simulink model "Simulation"  (R2019a)
settings: Solver=ode4  StartTime=0.0  StopTime=10  FixedStep=Ts  RelTol=1e-3
values from neighbouring files (symbols this model uses):
  B = (A'*A)\(A'*(Km*I)')    [Parametros_motor.m]
  J = M*R_rueda^2    (= 0.002772225)    [Parametros_motor.m]
  K = lqr(A_mat,B_mat,Q,R_mat)    [Parametros_motor.m]
  Ke = Ke'    [Parametros_motor.m]
  Km = (A'*A)\(A'*E')    [Parametros_motor.m]
  L = 2.04e-3    (= 0.00204)    [Parametros_motor.m]
  R = 5.06    [Parametros_motor.m]
  Ts = 1e-5    (= 1e-05)    [Parametros_motor.m]
  Tsc = 1e-3    (= 0.001)    [Parametros_motor.m]
  Tsco = 1e-3    (= 0.001)    [Parametros_motor.m]
undefined symbols (not defined in the file or in its folder): DiscIntNeverNeededParam
settings Model: SimulationMode=accelerator  Creator=cordo  LastModifiedBy=User

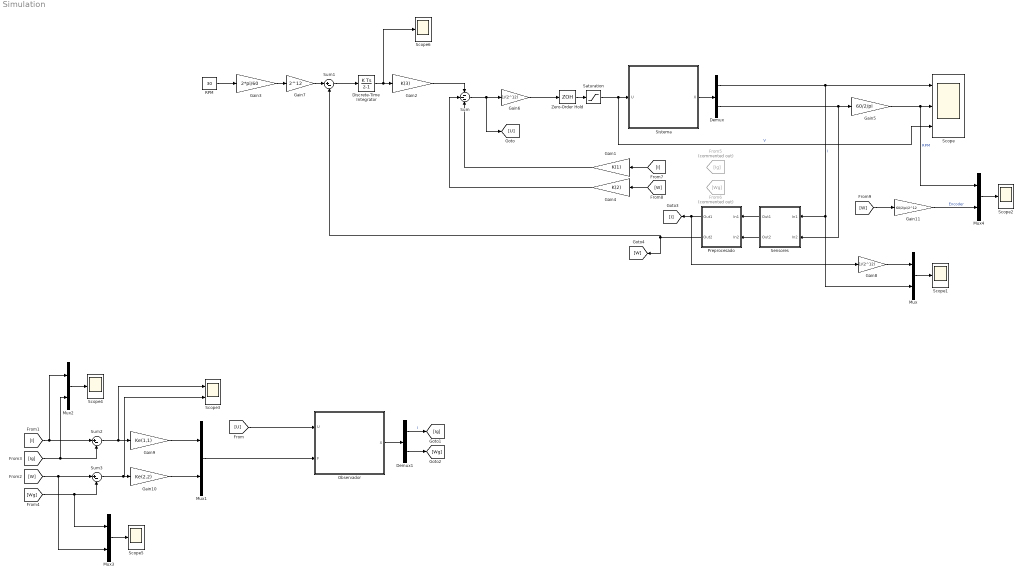
== system Simulation ==
  Demux : Demux  Outputs=2
  Demux1 : Demux  Outputs=2
  Discrete-Time Integrator : DiscreteIntegrator  SampleTime=Tsc  ICPrevOutput=DiscIntNeverNeededParam  ICPrevScaledInput=DiscIntNeverNeededParam
  From5 : From  Commented=on  GotoTag=Ig
  From6 : From  Commented=on  GotoTag=Wg
  Gain1 : Gain  Gain=K(1)
  Gain10 : Gain  Gain=Ke(2,2)
  Gain11 : Gain  Gain=60/2/pi/2^12
  Gain2 : Gain  Gain=K(3)
  Gain3 : Gain  Gain=2*pi/60
  Gain4 : Gain  Gain=K(2)
  Gain5 : Gain  Gain=60/2/pi
  Gain6 : Gain  Gain=1/(2^12)
  Gain7 : Gain  Gain=2^12
  Gain8 : Gain  Gain=1/(2^12)
  Gain9 : Gain  Gain=Ke(1,1)
  Mux{,1..4} (5 alike) : Mux  Inputs=2
  Observador : Subsystem
  Preprocesado : Subsystem
  RPM : Constant  Value=30  SampleTime=Ts
  Saturation : Saturate  UpperLimit=12.8  LowerLimit=-12.8
  Scope : Scope  NumInputPorts=3
  Scope{1..2,4..6} (5 alike) : Scope
  Scope3 : Scope  NumInputPorts=2
  Sensores : Subsystem
  Sistema : Subsystem
  Sum : Sum  Inputs=---
  Sum1 : Sum  Inputs=|+-
  Sum2 : Sum  Inputs=|+-
  Sum3 : Sum  Inputs=|+-
  Zero-Order Hold : ZeroOrderHold  SampleTime=Tsc
  wires:
  Sistema/1(X) -> Demux/1
  Demux/2 -> Sensores/2(In2), Gain5/1
  Demux/1 -> Mux/2, Sensores/1(In1), Scope/1  "I"
  Discrete-Time Integrator/1 -> Scope6/1, Gain2/1
  Gain4/1 -> Sum/2
  Gain3/1 -> Gain7/1
  RPM/1 -> Gain3/1
  Gain2/1 -> Sum/1
  Gain5/1 -> Mux4/1, Scope/2  "RPM"
  Sum/1 -> [U], Gain6/1
  Zero-Order Hold/1 -> Saturation/1
  Saturation/1 -> Scope/3, Sistema/1(U)  "V"
  Sum1/1 -> Discrete-Time Integrator/1
  Sensores/1(Out1) -> Preprocesado/1(In1)
  Sensores/2(Out2) -> Preprocesado/2(In2)
  Mux/1 -> Scope1/1
  Preprocesado/1(Out1) -> [I], Gain8/1
  Preprocesado/2(Out2) -> Sum1/2, [W]
  Gain6/1 -> Zero-Order Hold/1
  Gain7/1 -> Sum1/1
  Gain8/1 -> Mux/1
  Mux1/1 -> Observador/2(F)
  Gain9/1 -> Mux1/1
  Gain10/1 -> Mux1/2
  Observador/1(X) -> Demux1/1
  Demux1/1 -> [Ig]  "I"
  Demux1/2 -> [Wg]
  Sum2/1 -> Scope3/1, Gain9/1
  [I] -> Mux2/1, Sum2/1
  Sum3/1 -> Scope3/2, Gain10/1
  [Ig] -> Mux2/2, Sum2/2
  [Wg] -> Mux3/1, Sum3/2
  [U] -> Observador/1(U)
  Mux2/1 -> Scope4/1
  Mux3/1 -> Scope5/1
  [W] -> Mux3/2, Sum3/1
  [I] -> Gain1/1
  [W] -> Gain4/1
  Mux4/1 -> Scope2/1
  [W] -> Gain11/1
  Gain11/1 -> Mux4/2  "Encoder"
  Gain1/1 -> Sum/3

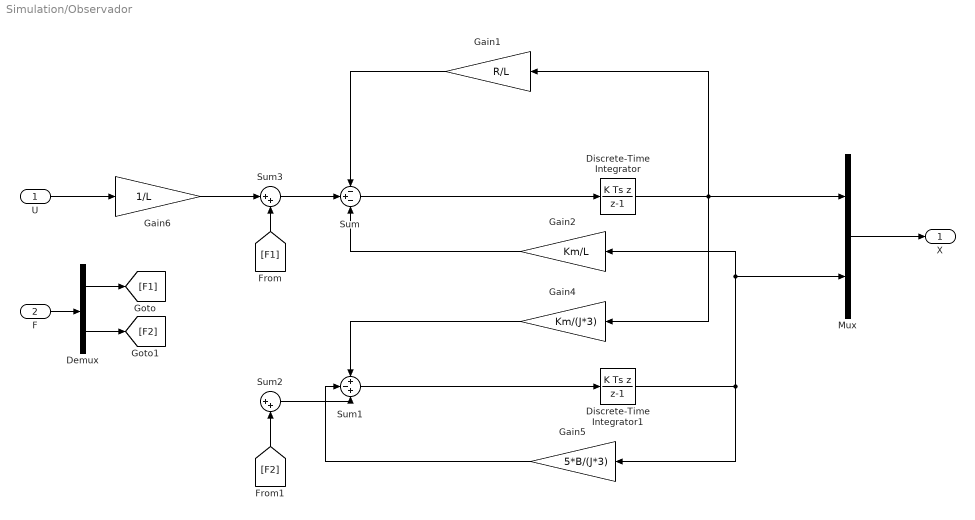
== system Simulation/Observador ==
  U : Inport
  F : Inport  Port=2
  Demux : Demux  Outputs=2
  Discrete-Time Integrator : DiscreteIntegrator  IntegratorMethod=Integration: Backward Euler  SampleTime=Tsco  ICPrevOutput=DiscIntNeverNeededParam  ICPrevScaledInput=DiscIntNeverNeededParam
  Discrete-Time Integrator1 : DiscreteIntegrator  IntegratorMethod=Integration: Backward Euler  SampleTime=Tsco  ICPrevOutput=DiscIntNeverNeededParam  ICPrevScaledInput=DiscIntNeverNeededParam
  Gain1 : Gain  Gain=R/L
  Gain2 : Gain  Gain=Km/L
  Gain4 : Gain  Gain=Km/(J*3)
  Gain5 : Gain  Gain=5*B/(J*3)
  Gain6 : Gain  Gain=1/L
  Mux : Mux  Inputs=2
  Sum : Sum  Inputs=-+-
  Sum1 : Sum  Inputs=+-+
  Sum2 : Sum  Inputs=|++
  Sum3 : Sum  Inputs=|++
  X : Outport
  wires:
  U/1 -> Gain6/1
  Mux/1 -> X/1
  Discrete-Time Integrator/1 -> Mux/1, Gain4/1, Gain1/1
  Sum1/1 -> Discrete-Time Integrator1/1
  Discrete-Time Integrator1/1 -> Mux/2, Gain2/1, Gain5/1
  Sum/1 -> Discrete-Time Integrator/1
  Gain2/1 -> Sum/3
  Gain4/1 -> Sum1/1
  Gain1/1 -> Sum/1
  Gain5/1 -> Sum1/2
  Sum2/1 -> Sum1/3
  Sum3/1 -> Sum/2
  Gain6/1 -> Sum3/1
  F/1 -> Demux/1
  Demux/1 -> [F1]
  [F1] -> Sum3/2
  Demux/2 -> [F2]
  [F2] -> Sum2/2

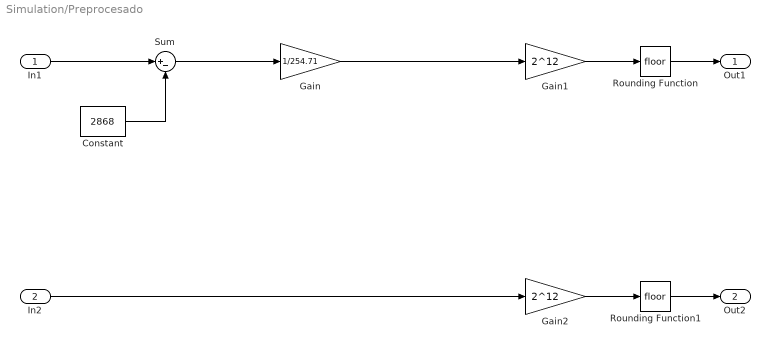
== system Simulation/Preprocesado ==
  In1 : Inport
  In2 : Inport  Port=2
  Constant : Constant  Value=2868
  Gain : Gain  Gain=1/254.71
  Gain1 : Gain  Gain=2^12
  Gain2 : Gain  Gain=2^12
  Rounding Function : Rounding
  Rounding Function1 : Rounding
  Sum : Sum  Inputs=|+-
  Out1 : Outport
  Out2 : Outport  Port=2
  wires:
  In2/1 -> Gain2/1
  Constant/1 -> Sum/2
  Sum/1 -> Gain/1
  In1/1 -> Sum/1
  Gain/1 -> Gain1/1
  Gain1/1 -> Rounding Function/1
  Gain2/1 -> Rounding Function1/1
  Rounding Function/1 -> Out1/1
  Rounding Function1/1 -> Out2/1

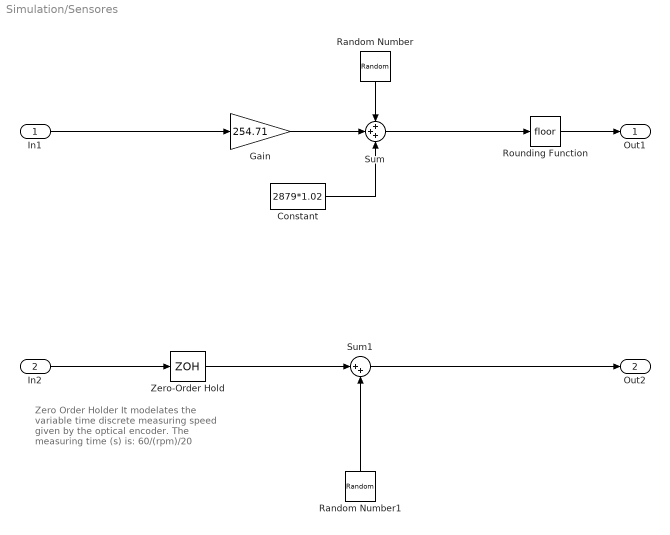
== system Simulation/Sensores ==
  note: Zero Order Holder
      | It modelates the variable time discrete
      | measuring  speed given by the optical
      | encoder.
      |
      | The measuring time (s) is:
      |
      | 60/(rpm)/20
  In1 : Inport
  In2 : Inport  Port=2
  Constant : Constant  Value=2879*1.02
  Gain : Gain  Gain=254.71
  Random Number : RandomNumber  Variance=20^2  SampleTime=Tsc
  Random Number1 : RandomNumber  Variance=4  SampleTime=Tsc
  Rounding Function : Rounding
  Sum : Sum  Inputs=+++
  Sum1 : Sum  Inputs=|++
  Zero-Order Hold : ZeroOrderHold  SampleTime=60/30/20
  Out1 : Outport
  Out2 : Outport  Port=2
  wires:
  Sum/1 -> Rounding Function/1
  In1/1 -> Gain/1
  Random Number/1 -> Sum/1
  Constant/1 -> Sum/3
  Gain/1 -> Sum/2
  Rounding Function/1 -> Out1/1
  In2/1 -> Zero-Order Hold/1
  Sum1/1 -> Out2/1
  Random Number1/1 -> Sum1/2
  Zero-Order Hold/1 -> Sum1/1

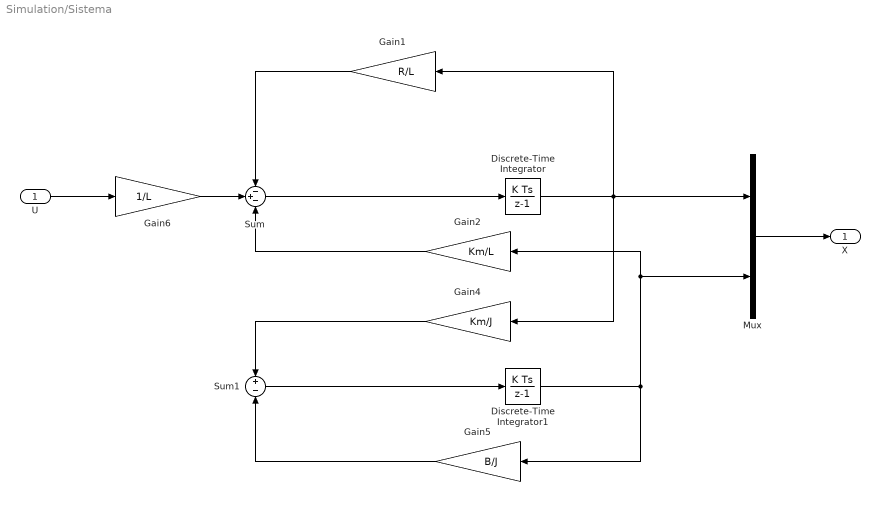
== system Simulation/Sistema ==
  U : Inport
  Discrete-Time Integrator : DiscreteIntegrator  SampleTime=Ts  ICPrevOutput=DiscIntNeverNeededParam  ICPrevScaledInput=DiscIntNeverNeededParam
  Discrete-Time Integrator1 : DiscreteIntegrator  SampleTime=Ts  ICPrevOutput=DiscIntNeverNeededParam  ICPrevScaledInput=DiscIntNeverNeededParam
  Gain1 : Gain  Gain=R/L
  Gain2 : Gain  Gain=Km/L
  Gain4 : Gain  Gain=Km/J
  Gain5 : Gain  Gain=B/J
  Gain6 : Gain  Gain=1/L
  Mux : Mux  Inputs=2
  Sum : Sum  Inputs=-+-
  Sum1 : Sum  Inputs=+-
  X : Outport
  wires:
  U/1 -> Gain6/1
  Mux/1 -> X/1
  Discrete-Time Integrator/1 -> Mux/1, Gain4/1, Gain1/1
  Sum1/1 -> Discrete-Time Integrator1/1
  Discrete-Time Integrator1/1 -> Mux/2, Gain2/1, Gain5/1
  Sum/1 -> Discrete-Time Integrator/1
  Gain2/1 -> Sum/3
  Gain4/1 -> Sum1/1
  Gain1/1 -> Sum/1
  Gain5/1 -> Sum1/2
  Gain6/1 -> Sum/2
